simulink model "exercise5Q3"  (R2023b)
settings: Solver=VariableStepAuto  StartTime=0.0  StopTime=10.0  RelTol=1e-3
undefined symbols (not defined in the file or in its folder): Plant
settings Model: Creator=bengo  LastModifiedBy=bengo

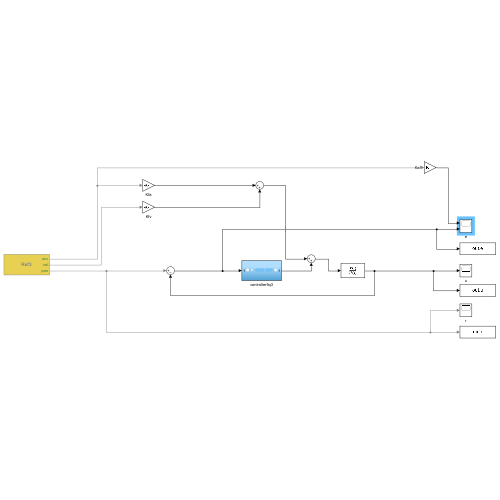
[thumbnail: Simulink's stored preview of the top-level diagram]
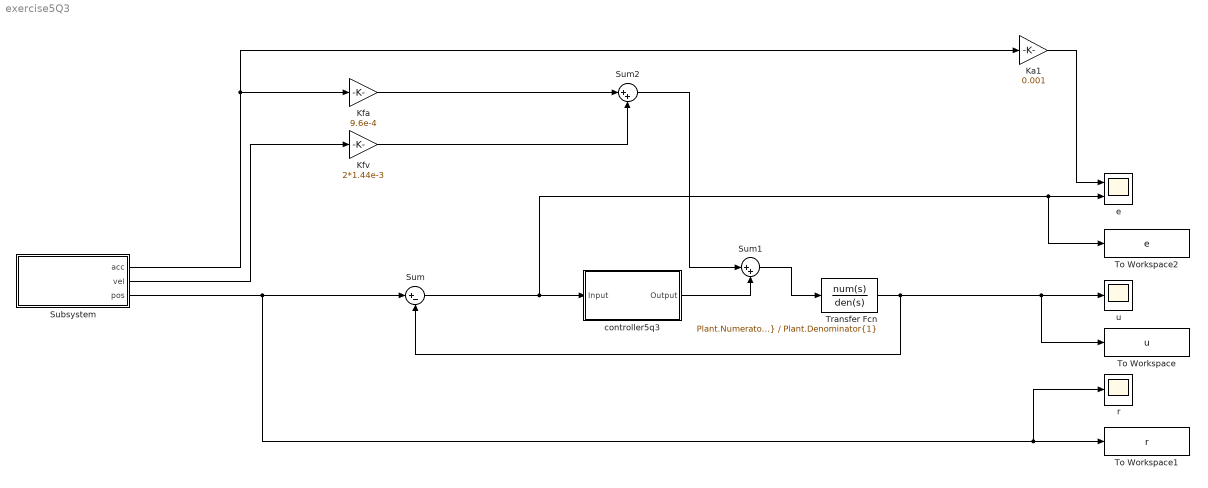
== system exercise5Q3 ==
  Ka1 : Gain  Gain=0.001
  Kfa : Gain  Gain=9.6e-4
  Kfv : Gain  Gain=2*1.44e-3
  Subsystem : Subsystem  mask(Ref3){}
      settings: OpenFcn=r3g_main
      mask Display: disp('Ref3');
  Sum : Sum  Inputs=|+-
  Sum1 : Sum  Inputs=|++
  Sum2 : Sum  Inputs=|++
  To Workspace : ToWorkspace  VariableName=u  SaveFormat=Timeseries  SampleTime=-1
  To Workspace1 : ToWorkspace  VariableName=r  SaveFormat=Timeseries  SampleTime=-1
  To Workspace2 : ToWorkspace  VariableName=e  SaveFormat=Timeseries  SampleTime=-1
  Transfer Fcn : TransferFcn  Numerator=Plant.Numerator{1}  Denominator=Plant.Denominator{1}
  controller5q3 : Subsystem
  e : Scope  NumInputPorts=2
  r : Scope
  u : Scope
  wires:
  Subsystem/3(pos) -> r/1, To Workspace1/1, Sum/1
  Transfer Fcn/1 -> To Workspace/1, u/1, Sum/2
  Subsystem/1(acc) -> Ka1/1, Kfa/1
  Sum/1 -> controller5q3/1(Input), To Workspace2/1, e/2
  Kfa/1 -> Sum2/1
  Ka1/1 -> e/1
  Subsystem/2(vel) -> Kfv/1
  Kfv/1 -> Sum2/2
  Sum2/1 -> Sum1/1
  Sum1/1 -> Transfer Fcn/1
  controller5q3/1(Output) -> Sum1/2

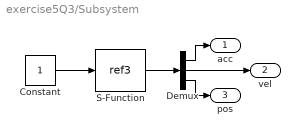
== system exercise5Q3/Subsystem ==
  Constant : Constant
  Demux : Demux  Outputs=3
      settings: DisplayOption=none
  S-Function : S-Function  FunctionName=ref3  Parameters=ref_part  SFunctionDeploymentMode=off  EnableBusSupport=off
      settings: OpenFcn=global ref_part; r3g_main
  acc : Outport
  vel : Outport  Port=2
  pos : Outport  Port=3
  wires:
  Constant/1 -> S-Function/1
  S-Function/1 -> Demux/1
  Demux/1 -> acc/1
  Demux/2 -> vel/1
  Demux/3 -> pos/1

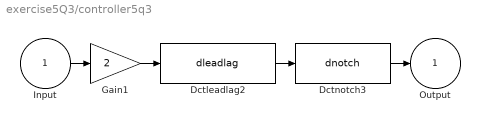
== system exercise5Q3/controller5q3 ==
  Input : Inport
  Dctleadlag2 : S-Function  FunctionName=dleadlag  Parameters=f_num, f_den, 0.001  SFunctionDeploymentMode=off  EnableBusSupport=off  mask(dctools){f_num=4, f_den=36}
      mask prompts: f_num "Zero [Hz]"; f_den "Pole [Hz]"
      mask help: This block implements a discrete time leadlag filter.
      mask Display: disp('DCT leadlag')
  Dctnotch3 : S-Function  FunctionName=dnotch  Parameters=f_num, b_num, f_den, b_den, 0.001  SFunctionDeploymentMode=off  EnableBusSupport=off  mask(dctools){f_num=47, b_num=0.02, f_den=47, b_den=0.5}
      mask prompts: f_num "Zero [Hz]"; b_num "Damping zero [-]"; f_den "Pole [Hz]"; b_den "Damping pole [-]"
      mask help: This block implements a dicrete time 2nd order notch filter.
      mask Display: disp('DCT notch')
  Gain1 : Gain  Gain=2
  Output : Outport
  wires:
  Input/1 -> Gain1/1
  Gain1/1 -> Dctleadlag2/1
  Dctleadlag2/1 -> Dctnotch3/1
  Dctnotch3/1 -> Output/1
